simulink model "accel_tc_sim"  (R2026a)
settings: Solver=FixedStepDiscrete  StopTime=7  FixedStep=0.0005
PreLoadFcn:
  | addpath(fullfile(fileparts(which('params_cfr26')),'lib'));
InitFcn:
  | addpath(fullfile(fileparts(which('params_cfr26')),'lib'));
settings Model: Creator=Aboud  LastModifiedBy=Aboud

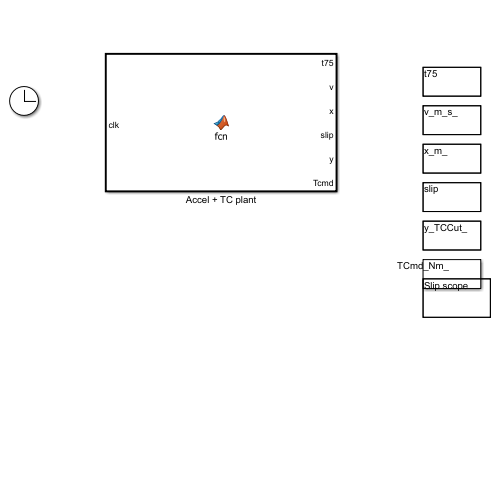
[thumbnail: Simulink's stored preview of the top-level diagram]
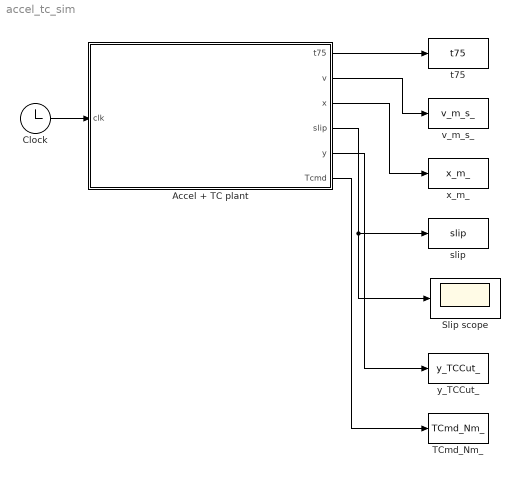
== system accel_tc_sim ==
  Accel + TC plant : MATLAB Function  TreatAsAtomicUnit=on
  Clock : Clock
  Slip scope : Scope
  TCmd_Nm_ : ToWorkspace  VariableName=TCmd_Nm_  SaveFormat=Structure With Time  SampleTime=-1
  slip : ToWorkspace  VariableName=slip  SaveFormat=Structure With Time  SampleTime=-1
  t75 : ToWorkspace  VariableName=t75  SaveFormat=Structure With Time  SampleTime=-1
  v_m_s_ : ToWorkspace  VariableName=v_m_s_  SaveFormat=Structure With Time  SampleTime=-1
  x_m_ : ToWorkspace  VariableName=x_m_  SaveFormat=Structure With Time  SampleTime=-1
  y_TCCut_ : ToWorkspace  VariableName=y_TCCut_  SaveFormat=Structure With Time  SampleTime=-1
  wires:
  Clock/1 -> Accel + TC plant/1(clk)
  Accel + TC plant/3(x) -> x_m_/1
  Accel + TC plant/2(v) -> v_m_s_/1
  Accel + TC plant/1(t75) -> t75/1
  Accel + TC plant/6(Tcmd) -> TCmd_Nm_/1
  Accel + TC plant/4(slip) -> slip/1, Slip scope/1
  Accel + TC plant/5(y) -> y_TCCut_/1

== matlab function accel_tc_sim/Accel + TC plant ==
  data: t75 output; v output; x output; slip output; clk input; y output; Tcmd output
function [t75, v, x, slip, y, Tcmd] = fcn(clk)
% Thin wrapper. All physics + control live in lib/accel_tc_core.m, called
% through lib/accel_tc_sample.m, so Simulink and accel_model_tc.m can never
% disagree -- there is one implementation, and both call it.
coder.extrinsic('accel_tc_sample');
t75 = 0; v = 0; x = 0; slip = 0; y = 0; Tcmd = 0;
[t75, v, x, slip, y, Tcmd] = accel_tc_sample(clk);
